simulink library "ProductionLineLib_CM"  (R2024b)
settings: Solver=VariableStepAuto  StartTime=0.0  StopTime=10.0  RelTol=1e-3
libraries: NSA_DEVS_MATH_OPERATIONS x70, $bdroot x37, NSA_DEVS_SOURCES x23, ProductionLineLib_AM x7, NSA_DEVS_DIGITAL_CONVERTER x6, NSA_DEVS_STATISTICS x5, NSA_DEVS_QSS x5, NSA_DEVS_ROUTING x4, NSA_DEVS_LOGISTICS x3, NSA_DEVS_DIGITAL_LOGIC x2
(part 2 of 2)

== system ProductionLineLib_CM/turningPowerSupply ==
  turning : Inport
  on : Inport  Port=2
  add2 : NSA_DEVS_MATH_OPERATIONS/am_add2  tau=[0,1]  debug=debug
      settings: SourceProductName=Math Operations
  const : NSA_DEVS_SOURCES/am_const  value=vcc_load  sendTime=[0,1]  debug=debug
      settings: SourceProductName=Sources
  const1 : NSA_DEVS_SOURCES/am_const  value=vcc  sendTime=[0,1]  debug=debug
      settings: SourceProductName=Sources
  multi1 : NSA_DEVS_MATH_OPERATIONS/am_mult2  tau=tau  debug=debug
      settings: SourceProductName=Math Operations
  multi2 : NSA_DEVS_MATH_OPERATIONS/am_mult2  tau=[0,1]  debug=debug
      settings: SourceProductName=Math Operations
  u : Outport
  wires:
  const1/1 -> add2/1
  turning/1 -> multi1/1
  const/1 -> multi1/2
  multi2/1 -> u/1
  on/1 -> multi2/2
  add2/1 -> multi2/1
  multi1/1 -> add2/2

== system ProductionLineLib_CM/turning_CM ==
  entered : Inport
  ap : Inport  Port=2
  f : Inport  Port=3
  vc : Inport  Port=4
  turning_controller1 : ProductionLineLib_AM/turning_controller  turning_time=turning_time  ap_ug=ap_ug  f_ug=f_ug  vc_ug=vc_ug  ap_og=ap_og  f_og=f_og  vc_og=vc_og  tau=tau  debug=debug
  on : Outport
  turning : Outport  Port=2
  phase : Outport  Port=3
  leaving : Outport  Port=4
  wires:
  vc/1 -> turning_controller1/4
  f/1 -> turning_controller1/3
  ap/1 -> turning_controller1/2
  turning_controller1/3 -> phase/1
  turning_controller1/2 -> turning/1
  turning_controller1/1 -> on/1
  entered/1 -> turning_controller1/1
  turning_controller1/4 -> leaving/1

== system ProductionLineLib_CM/turning_PM ==
  on : Inport
  turning : Inport  Port=2
  ap : Inport  Port=3
  f : Inport  Port=4
  vc : Inport  Port=5
  turningMotorI : $bdroot/turningMotorI  R=R  L=L  K=K  tauInt=tauInt  tau=[0,1]  debug=debug
  turningMotorN : $bdroot/turningMotorN  J=J  b=b  K=K  load=load  tauInt=tauInt  tau=[0,1]  debug=debug
  turningPfCalc : $bdroot/turningPfCalc  ap_ug=ap_ug  ap_og=ap_og  P_ap=P_ap  f_ug=f_ug  f_og=f_og  P_f=P_f  vc_ug=vc_ug  vc_og=vc_og  P_vc=P_vc  tau=tau  debug=debug
  turningPowerCalc : $bdroot/turningPowerCalc  tauInt=tauInt  tau=[0,1]  debug=debug
  turningPowerSupply : $bdroot/turningPowerSupply  vcc=vcc  vcc_load=vcc_load  tau=tau  debug=debug
  e : Outport
  u : Outport  Port=2
  p : Outport  Port=3
  i : Outport  Port=4
  n : Outport  Port=5
  wires:
  ap/1 -> turningPfCalc/1
  f/1 -> turningPfCalc/2
  vc/1 -> turningPfCalc/3
  turning/1 -> turningMotorN/2, turningPowerSupply/1, turningPfCalc/4
  turningPfCalc/1 -> turningPowerCalc/1
  turningPowerCalc/1 -> i/1
  turningPowerCalc/2 -> p/1
  turningPowerCalc/3 -> e/1
  turningMotorI/1 -> turningMotorN/1, turningPowerCalc/3
  turningMotorN/1 -> n/1
  turningMotorN/2 -> turningMotorI/2
  turningPowerSupply/1 -> turningMotorI/1, turningPowerCalc/2, u/1
  on/1 -> turningPowerSupply/2
